simulink model "untitled1"  (R2020a)
settings: Solver=VariableStepAuto  StartTime=0.0  StopTime=inf  RelTol=1e-3
undefined symbols (not defined in the file): IMU_sensor, left_motor, motors, right_motor, TIME_STEP
libraries: simulink x2
settings Model: Creator=Vulca  LastModifiedBy=Vulca

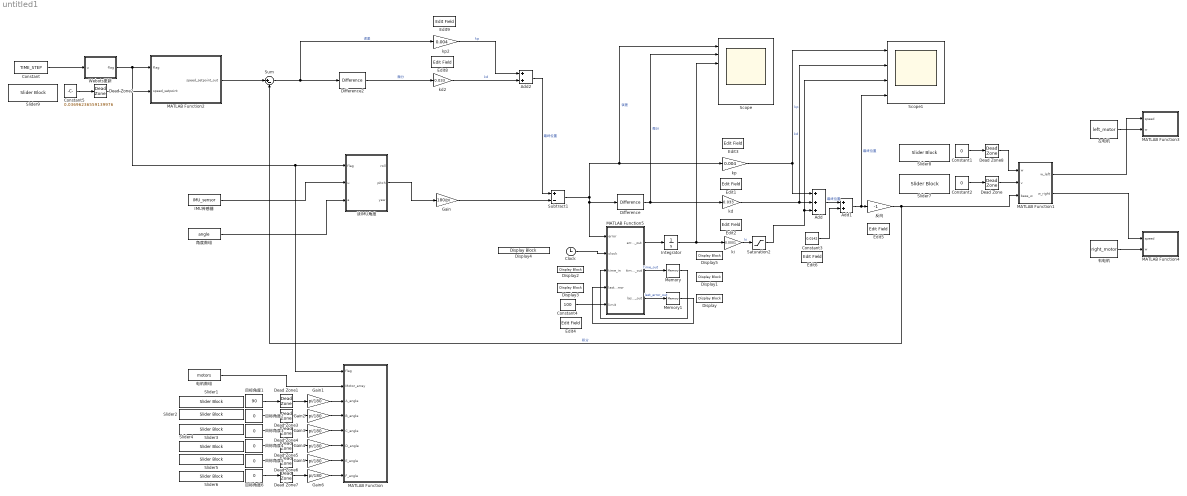
== system untitled1 ==
  Add : Sum  Inputs=+++
  Add1 : Sum
  Add2 : Sum
  Clock : Clock
  Constant : Constant  Value=TIME_STEP
  Constant1 : Constant  Value=0
  Constant2 : Constant  Value=0
  Constant3 : Constant  Value=0.0142
  Constant4 : Constant  Value=100
  Constant5 : Constant  Value=0.03696236559139976
  Dead Zone{,1,3..7} (7 alike) : DeadZone  LowerValue=-2  UpperValue=2  SaturateOnIntegerOverflow=on
  Dead Zone2 : DeadZone  SaturateOnIntegerOverflow=on
  Dead Zone8 : DeadZone  SaturateOnIntegerOverflow=on
  Difference : simulink/Discrete/Difference  ICPrevInput=0.0  OutMin=[]  OutMax=[]  OutDataType=fixdt(1, 16)  OutScaling=2^-10  DoSatur=off
  Difference2 : simulink/Discrete/Difference  ICPrevInput=0.0  OutMin=[]  OutMax=[]  OutDataType=fixdt(1, 16)  OutScaling=2^-10  DoSatur=off
  Display{,1..5} (6 alike) : DisplayBlock  LabelPosition=Hide  Format=short  Transparency=1
  Edit{1..6,8..9} (8 alike) : EditField  LabelPosition=Hide  ShowInitialText=on  Alignment=Center
  Gain : Gain  Gain=180/pi
  Gain{1..6} (6 alike) : Gain  Gain=pi/180
  IMU传感器 : Constant  Value=IMU_sensor
  Integrator : Integrator
  MATLAB Function : MATLAB Function  TreatAsAtomicUnit=on
  MATLAB Function1 : MATLAB Function  TreatAsAtomicUnit=on
  MATLAB Function2 : MATLAB Function  TreatAsAtomicUnit=on
  MATLAB Function3 : MATLAB Function  TreatAsAtomicUnit=on
  MATLAB Function4 : MATLAB Function  TreatAsAtomicUnit=on
  MATLAB Function5 : MATLAB Function  TreatAsAtomicUnit=on
  Memory : Memory
  Memory1 : Memory
  Saturation2 : Saturate  UpperLimit=0.1  LowerLimit=-0.1
  Scope : Scope  NumInputPorts=7
  Scope1 : Scope  NumInputPorts=4
  Slider{1..6} (6 alike) : SliderBlock  ScaleMin=-180  ScaleMax=180
  Slider7 : SliderBlock  ScaleMin=-20  ScaleMax=20
  Slider8 : SliderBlock  ScaleMin=-20  ScaleMax=20
  Slider9 : SliderBlock  ScaleMin=-20  ScaleMax=20
  Subtract1 : Sum  Inputs=+-
  Sum : Sum  Inputs=|+-
  Webots更新 : MATLAB Function  TreatAsAtomicUnit=on
  kd : Gain  Gain=0.033
  kd2 : Gain  Gain=0.033
  ki : Gain  Gain=0.0001
  kp : Gain  Gain=0.004
  kp2 : Gain  Gain=0.004
  反向 : Gain  Gain=-1
  右电机 : Constant  Value=right_motor
  左电机 : Constant  Value=left_motor
  电机数组 : Constant  Value=motors
  目标角度1 : Constant  Value=90
  目标角度{2..6} (5 alike) : Constant  Value=0
  角度数组 : Constant  Value=angle
  读IMU角度 : MATLAB Function  TreatAsAtomicUnit=on
  wires:
  Integrator/1 -> Scope/3, ki/1
  Constant1/1 -> Dead Zone8/1
  Add/1 -> Add1/1  "最终位置"
  Constant2/1 -> Dead Zone/1
  MATLAB Function1/1(w_left) -> MATLAB Function3/1(speed)
  MATLAB Function1/2(w_right) -> MATLAB Function4/1(speed)
  右电机/1 -> MATLAB Function4/2(w)
  左电机/1 -> MATLAB Function3/2(w)
  Dead Zone5/1 -> Gain4/1
  Subtract1/1 -> kp/1, Scope/1, MATLAB Function5/1(error), Difference/1  "误差"
  Dead Zone4/1 -> Gain3/1
  Dead Zone7/1 -> Gain6/1
  Gain2/1 -> MATLAB Function/4(B_angle)
  Gain3/1 -> MATLAB Function/5(C_angle)
  读IMU角度/2(pitch) -> Gain/1
  目标角度3/1 -> Dead Zone4/1
  Gain1/1 -> MATLAB Function/3(A_angle)
  电机数组/1 -> MATLAB Function/2(Motor_array)
  ki/1 -> Saturation2/1  "ki"
  kp/1 -> Scope1/1, Add/1  "kp"
  IMU传感器/1 -> 读IMU角度/2(u)
  Dead Zone1/1 -> Gain1/1
  Saturation2/1 -> Scope1/3, Add/3
  Dead Zone3/1 -> Gain2/1
  目标角度2/1 -> Dead Zone3/1
  Add1/1 -> Scope1/4, 反向/1  "最终位置"
  角度数组/1 -> 读IMU角度/3(a)
  Gain/1 -> Subtract1/2
  MATLAB Function5/3(last_error_out) -> Memory1/1  "last_error_out"
  MATLAB Function5/1(error_out) -> Integrator/1
  Dead Zone6/1 -> Gain5/1
  Gain5/1 -> MATLAB Function/7(E_angle)
  Gain6/1 -> MATLAB Function/8(F_angle)
  目标角度5/1 -> Dead Zone6/1
  Memory1/1 -> MATLAB Function5/4(last_error)
  Dead Zone8/1 -> MATLAB Function1/1(w)
  kd/1 -> Scope1/2, Add/2  "kd"
  目标角度6/1 -> Dead Zone7/1
  Memory/1 -> MATLAB Function5/3(time_in)
  Clock/1 -> MATLAB Function5/2(clock)
  Constant/1 -> Webots更新/1(u)
  Constant4/1 -> MATLAB Function5/5(limit)
  Difference/1 -> kd/1, Scope/2  "微分"
  Gain4/1 -> MATLAB Function/6(D_angle)
  MATLAB Function5/2(time_out) -> Memory/1  "time_out"
  目标角度4/1 -> Dead Zone5/1
  目标角度1/1 -> Dead Zone1/1
  Constant3/1 -> Add1/2
  Dead Zone/1 -> MATLAB Function1/2(v)
  反向/1 -> MATLAB Function1/3(base_w), Sum/2  "积分"
  Webots更新/1(flag) -> MATLAB Function/1(flag), 读IMU角度/1(flag), MATLAB Function2/1(flag)
  MATLAB Function2/1(speed_setpoint_out) -> Sum/1
  Difference2/1 -> kd2/1  "微分"
  kd2/1 -> Add2/2  "kd"
  Sum/1 -> kp2/1, Difference2/1  "误差"
  kp2/1 -> Add2/1  "kp"
  Add2/1 -> Subtract1/1  "最终位置"
  Constant5/1 -> Dead Zone2/1
  Dead Zone2/1 -> MATLAB Function2/2(speed_setpoint)

== matlab function untitled1/Webots更新 ==
  data: u input; flag output
function flag = fcn(u)
wb_robot_step(u);
flag = 1;

== matlab function untitled1/读IMU角度 ==
  data: flag input; u input; roll output; a input; pitch output; yaw output
function [roll,pitch,yaw] = fcn(flag,u,a)
roll = 0.0;
pitch = 0.0;
yaw = 0.0;
switch flag
    case 1
       a=wb_inertial_unit_get_roll_pitch_yaw(u);
end
roll = a(1);
pitch = a(2);
yaw = a(3);

== matlab function untitled1/MATLAB Function2 ==
  data: flag input; speed_setpoint input; speed_setpoint_out output
function speed_setpoint_out= fcn(flag,speed_setpoint)
speed_setpoint_out = speed_setpoint;

== matlab function untitled1/MATLAB Function ==
  data: flag input; Motor_array input; A_angle input; B_angle input; C_angle input; D_angle input; E_angle input; F_angle input
function fcn(flag,Motor_array,A_angle,B_angle,C_angle,D_angle,E_angle,F_angle)
switch flag
    case 1
        wb_motor_set_position(Motor_array(1),A_angle);
        wb_motor_set_position(Motor_array(2),B_angle);
        wb_motor_set_position(Motor_array(3),C_angle);
        wb_motor_set_position(Motor_array(4),D_angle);
        wb_motor_set_position(Motor_array(5),E_angle);
        wb_motor_set_position(Motor_array(6),F_angle);
end

== matlab function untitled1/MATLAB Function1 ==
  data: w input; w_left output; w_right output; v input; base_w input
function [w_left,w_right]= fcn(w,v,base_w)

w_left = v+w+base_w;
w_right = v-w+base_w;

== matlab function untitled1/MATLAB Function3 ==
  data: speed input; w input
function fcn(speed,w)
wb_motor_set_velocity(w,speed);

== matlab function untitled1/MATLAB Function4 ==
  data: speed input; w input
function fcn(speed,w)
wb_motor_set_velocity(w,speed);

== matlab function untitled1/MATLAB Function5 ==
  data: error_out output; time_out output; error input; clock input; time_in input; last_error input; limit input; last_error_out output
function [error_out,time_out,last_error_out] = fcn(error,clock,time_in,last_error,limit)

%判断误差是否过零点
if (last_error>=0 && error < 0) || (last_error <=0 && error > 0)
    %记录过零点时间
    time_out = clock;
else
    time_out = time_in;
end

%积分环节停止积分
error_out = 0;

%若距离上次error == 0 已经很长时间了
if (clock - time_in)>limit && abs(error)>0.5
    %启用积分环节
    error_out = error;
end
last_error_out = error;
